simulink model "part_n"  (R2022b)
settings: Solver=ode4  StartTime=0.0  StopTime=inf  FixedStep=0.002  RelTol=1e-3
InitFcn:
  | init; % init script
undefined symbols (not defined in the file or in its folder): attitude_m0, attitude_t0, d_state_m, d_state_t, k_epsilon_lead_angle, k_sigma_lead_angle, state_m0, state_t0
libraries: simulink x1
settings Model: SimulationMode=external  Creator=Ali  LastModifiedBy=Ali
settings HardwareCC: ProdBitPerLong=64  ProdHWDeviceType=Intel->x86-64 (Linux 64)
settings RTWCC: Description=Simulink Desktop Real-Time  SystemTargetFile=sldrt.tlc  TemplateMakefile=sldrt.tmf  RTWCompilerOptimization=on
settings CodeAppCC: MaxIdLength=95
settings SimulinkDesktopRealTimeCC: TargetLibSuffix=_sldrt.a  TargetPreCompLibLocation=/Applications/MATLAB_R2022b.app/toolbox/sldrt/lib/maci64

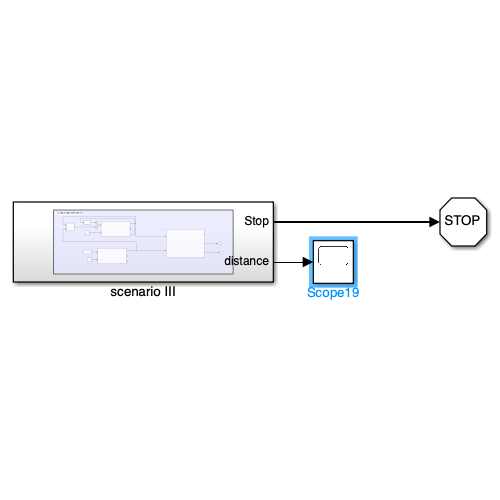
[thumbnail: Simulink's stored preview of the top-level diagram]
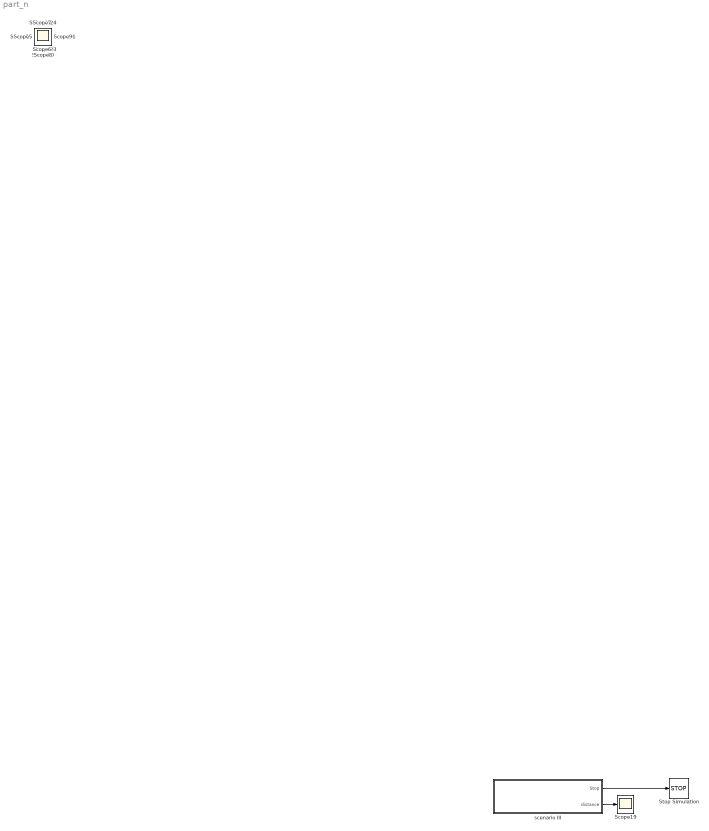
== system part_n ==
  Scope{,1..24} (25 alike) : Scope
  Stop Simulation : Stop
  scenario III : Subsystem
  wires:
  scenario III/1(Stop) -> Stop Simulation/1
  scenario III/2(distance) -> Scope19/1

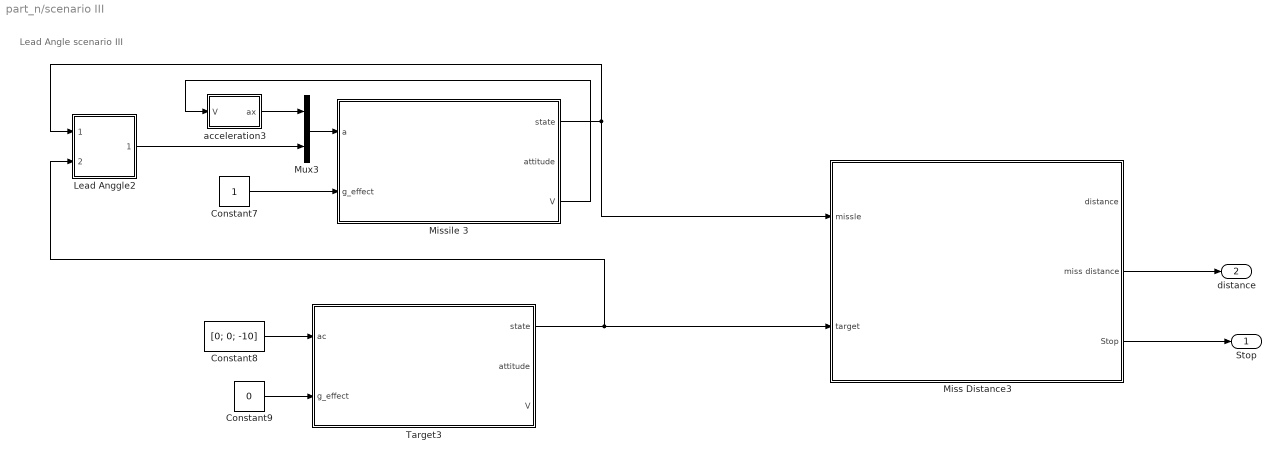
== system part_n/scenario III ==
  note: Lead Angle scenario III
  Constant7 : Constant
  Constant8 : Constant  Value=[0; 0; -10]
  Constant9 : Constant  Value=0
  Lead Anggle2 : Subsystem
  Miss Distance3 : Subsystem
  Missile 3 : Subsystem
  Mux3 : Mux  Inputs=2
  Target3 : Subsystem
  acceleration3 : Subsystem
  Stop : Outport
  distance : Outport  Port=2
  wires:
  Miss Distance3/3(Stop) -> Stop/1
  Target3/1(state) -> Lead Anggle2/2(target_state), Miss Distance3/2(target)
  acceleration3/1(ax) -> Mux3/1
  Lead Anggle2/1("ay, az") -> Mux3/2
  Missile 3/1(state) -> Lead Anggle2/1(missle_state), Miss Distance3/1(missle)
  Constant7/1 -> Missile 3/2(g_effect)
  Constant9/1 -> Target3/2(g_effect)
  Missile 3/3(V) -> acceleration3/1(V)
  Miss Distance3/2(miss distance) -> distance/1
  Constant8/1 -> Target3/1(ac)
  Mux3/1 -> Missile 3/1(a)

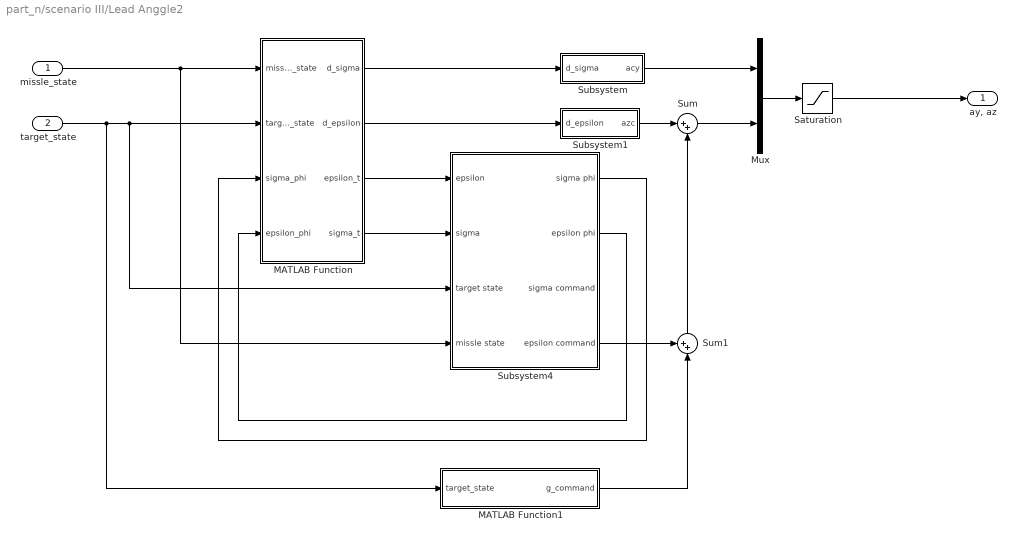
== system part_n/scenario III/Lead Anggle2 ==
  missle_state : Inport
  target_state : Inport  Port=2
  MATLAB Function : MATLAB Function  TreatAsAtomicUnit=on
  MATLAB Function1 : MATLAB Function  TreatAsAtomicUnit=on
  Mux : Mux  Inputs=2
  Saturation : Saturate  UpperLimit=5*9.81  LowerLimit=-5*9.81
  Subsystem : Subsystem
  Subsystem1 : Subsystem
  Subsystem4 : Subsystem
  Sum : Sum  Inputs=|++
  Sum1 : Sum  Inputs=++|
  "ay, az" : Outport
  wires:
  missle_state/1 -> Subsystem4/4(missle state), MATLAB Function/1(missle_state)
  target_state/1 -> MATLAB Function1/1(target_state), Subsystem4/3(target state), MATLAB Function/2(target_state)
  MATLAB Function/1(d_sigma) -> Subsystem/1(d_sigma)
  MATLAB Function/2(d_epsilon) -> Subsystem1/1(d_epsilon)
  Subsystem1/1(azc) -> Sum/1
  Mux/1 -> Saturation/1
  Saturation/1 -> "ay, az"/1
  Subsystem/1(acy) -> Mux/1
  Sum/1 -> Mux/2
  MATLAB Function/3(epsilon_t) -> Subsystem4/1(epsilon)
  MATLAB Function/4(sigma_t) -> Subsystem4/2(sigma)
  Subsystem4/1(sigma phi) -> MATLAB Function/3(sigma_phi)
  Subsystem4/2(epsilon phi) -> MATLAB Function/4(epsilon_phi)
  Sum1/1 -> Sum/2
  MATLAB Function1/1(g_command) -> Sum1/2
  Subsystem4/4(epsilon command) -> Sum1/1

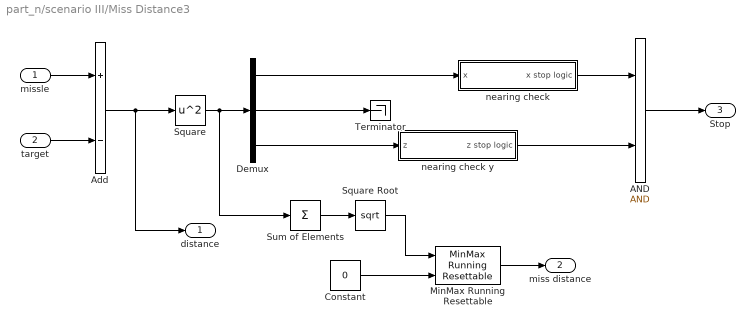
== system part_n/scenario III/Miss Distance3 ==
  missle : Inport
  target : Inport  Port=2
  AND : Logic  IconShape=distinctive  AllPortsSameDT=off  OutDataTypeStr=boolean
  Add : Sum  Inputs=+-
  Constant : Constant  Value=0
  Demux : Demux  Outputs=3
  MinMax Running Resettable : simulink/Math Operations/MinMax Running Resettable  Function=min  vinit=inf
  Square : Math  Operator=square
  Square Root : Sqrt
  Sum of Elements : Sum  Inputs=+
  Terminator : Terminator
  nearing check : Subsystem
  nearing check y : Subsystem
  distance : Outport
  miss distance : Outport  Port=2
  Stop : Outport  Port=3
  wires:
  missle/1 -> Add/1
  Add/1 -> distance/1, Square/1
  target/1 -> Add/2
  Square/1 -> Sum of Elements/1, Demux/1
  nearing check/1(x stop logic) -> AND/1
  AND/1 -> Stop/1
  Demux/2 -> Terminator/1
  nearing check y/1(z stop logic) -> AND/2
  Sum of Elements/1 -> Square Root/1
  Square Root/1 -> MinMax Running Resettable/1
  Demux/3 -> nearing check y/1(z)
  Demux/1 -> nearing check/1(x)
  Constant/1 -> MinMax Running Resettable/2
  MinMax Running Resettable/1 -> miss distance/1

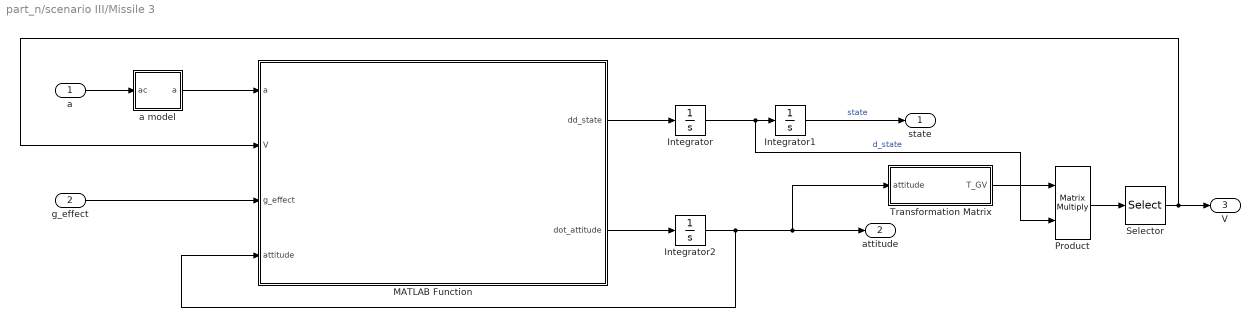
== system part_n/scenario III/Missile 3 ==
  a : Inport
  g_effect : Inport  Port=2
  Integrator : Integrator  InitialCondition=d_state_m
  Integrator1 : Integrator  InitialCondition=state_m0
  Integrator2 : Integrator  InitialCondition=attitude_m0
  MATLAB Function : MATLAB Function  TreatAsAtomicUnit=on
  Product : Product  Multiplication=Matrix(*)
  Selector : Selector  InputPortWidth=3  IndexOptions=Index vector (dialog)  Indices=[1]  OutputSizes=1
  Transformation Matrix : MATLAB Function  TreatAsAtomicUnit=on
  a model : Subsystem
  state : Outport
  attitude : Outport  Port=2
  V : Outport  Port=3
  wires:
  MATLAB Function/2(dot_attitude) -> Integrator2/1
  Integrator1/1 -> state/1  "state"
  MATLAB Function/1(dd_state) -> Integrator/1
  g_effect/1 -> MATLAB Function/3(g_effect)
  Integrator/1 -> Product/2, Integrator1/1  "d_state"
  Product/1 -> Selector/1
  Selector/1 -> MATLAB Function/2(V), V/1
  Transformation Matrix/1(T_GV) -> Product/1
  Integrator2/1 -> Transformation Matrix/1(attitude), attitude/1, MATLAB Function/4(attitude)
  a/1 -> a model/1(ac)
  a model/1(a) -> MATLAB Function/1(a)

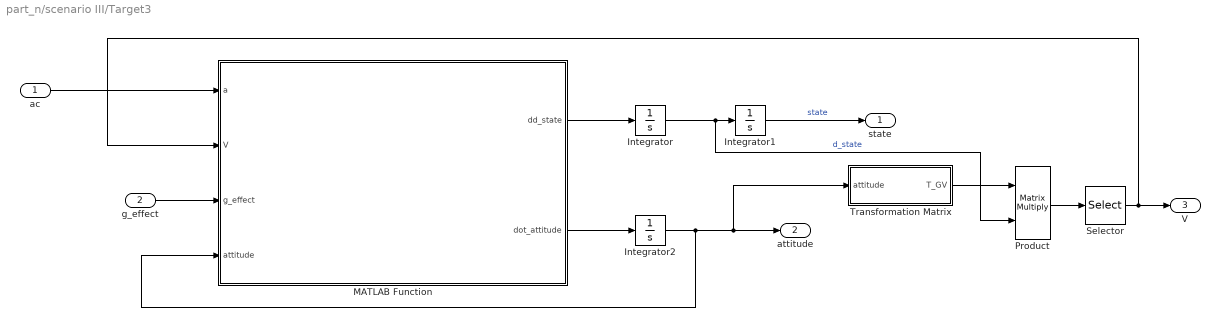
== system part_n/scenario III/Target3 ==
  ac : Inport
  g_effect : Inport  Port=2
  Integrator : Integrator  InitialCondition=d_state_t
  Integrator1 : Integrator  InitialCondition=state_t0
  Integrator2 : Integrator  InitialCondition=attitude_t0
  MATLAB Function : MATLAB Function  TreatAsAtomicUnit=on
  Product : Product  Multiplication=Matrix(*)
  Selector : Selector  InputPortWidth=3  IndexOptions=Index vector (dialog)  Indices=[1]  OutputSizes=1
  Transformation Matrix : MATLAB Function  TreatAsAtomicUnit=on
  state : Outport
  attitude : Outport  Port=2
  V : Outport  Port=3
  wires:
  MATLAB Function/2(dot_attitude) -> Integrator2/1
  Integrator1/1 -> state/1  "state"
  MATLAB Function/1(dd_state) -> Integrator/1
  g_effect/1 -> MATLAB Function/3(g_effect)
  Integrator/1 -> Product/2, Integrator1/1  "d_state"
  Integrator2/1 -> MATLAB Function/4(attitude), Transformation Matrix/1(attitude), attitude/1
  Product/1 -> Selector/1
  Selector/1 -> MATLAB Function/2(V), V/1
  Transformation Matrix/1(T_GV) -> Product/1
  ac/1 -> MATLAB Function/1(a)

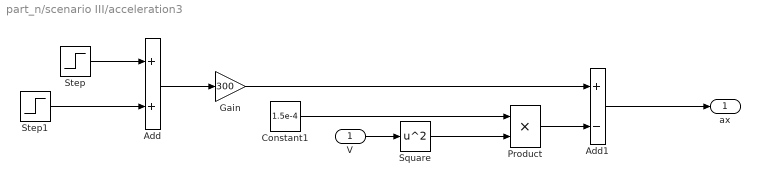
== system part_n/scenario III/acceleration3 ==
  V : Inport
  Add : Sum
  Add1 : Sum  Inputs=+-
  Constant1 : Constant  Value=1.5e-4
  Gain : Gain  Gain=300
  Product : Product
  Square : Math  Operator=square
  Step : Step  Time=3  After=-1  SampleTime=0
  Step1 : Step  Time=0  SampleTime=0
  ax : Outport
  wires:
  V/1 -> Square/1
  Step/1 -> Add/1
  Square/1 -> Product/2
  Constant1/1 -> Product/1
  Add1/1 -> ax/1
  Step1/1 -> Add/2
  Gain/1 -> Add1/1
  Add/1 -> Gain/1
  Product/1 -> Add1/2

== system part_n/scenario III/Lead Anggle2/Subsystem ==
  d_sigma : Inport
  Gain : Gain  Gain=k_sigma_lead_angle
  Sum : Sum  Inputs=+|+
  Transfer Fcn : TransferFcn  Numerator=[1000 0]  Denominator=[1 100]
  acy : Outport
  wires:
  d_sigma/1 -> Gain/1, Transfer Fcn/1
  Transfer Fcn/1 -> Sum/2
  Sum/1 -> acy/1
  Gain/1 -> Sum/1

== system part_n/scenario III/Lead Anggle2/Subsystem1 ==
  d_epsilon : Inport
  Gain1 : Gain  Gain=k_epsilon_lead_angle
  Sum : Sum  Inputs=+|+
  Transfer Fcn : TransferFcn  Numerator=[1000 0]  Denominator=[1 100]
  azc : Outport
  wires:
  d_epsilon/1 -> Transfer Fcn/1, Gain1/1
  Gain1/1 -> Sum/1
  Transfer Fcn/1 -> Sum/2
  Sum/1 -> azc/1

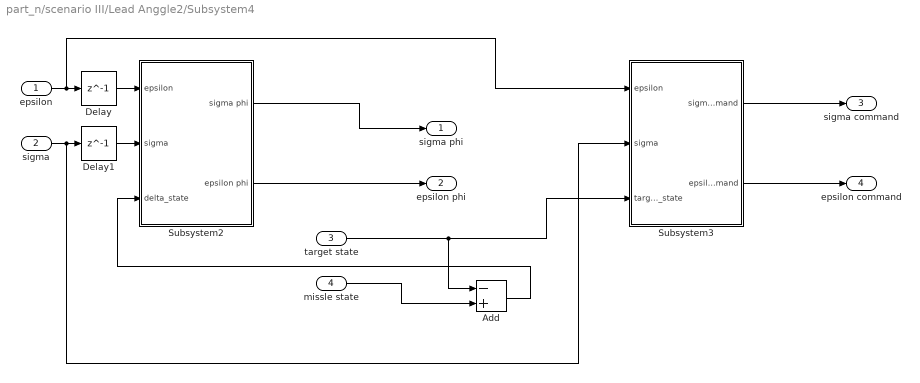
== system part_n/scenario III/Lead Anggle2/Subsystem4 ==
  epsilon : Inport
  sigma : Inport  Port=2
  target state : Inport  Port=3
  missle state : Inport  Port=4
  Add : Sum  Inputs=-+
  Delay : Delay  DelayLength=1
  Delay1 : Delay  DelayLength=1
  Subsystem2 : Subsystem
  Subsystem3 : Subsystem
  sigma phi : Outport
  epsilon phi : Outport  Port=2
  sigma command : Outport  Port=3
  epsilon command : Outport  Port=4
  wires:
  sigma/1 -> Subsystem3/2(sigma), Delay1/1
  epsilon/1 -> Subsystem3/1(epsilon), Delay/1
  Delay1/1 -> Subsystem2/2(sigma)
  Delay/1 -> Subsystem2/1(epsilon)
  Subsystem2/2(epsilon phi) -> epsilon phi/1
  Subsystem2/1(sigma phi) -> sigma phi/1
  target state/1 -> Add/1, Subsystem3/3(target_state)
  missle state/1 -> Add/2
  Add/1 -> Subsystem2/3(delta_state)
  Subsystem3/1(sigma command) -> sigma command/1
  Subsystem3/2(epsilon command) -> epsilon command/1

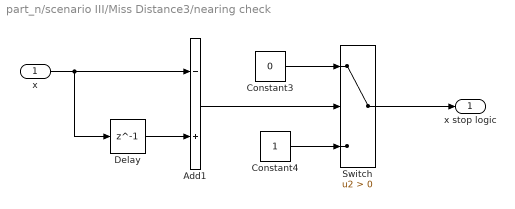
== system part_n/scenario III/Miss Distance3/nearing check ==
  x : Inport
  Add1 : Sum  Inputs=-+
  Constant3 : Constant  Value=0
  Constant4 : Constant
  Delay : Delay  DelayLength=1  InitialCondition=inf
  Switch : Switch  Criteria=u2 > Threshold  SaturateOnIntegerOverflow=off  InputSameDT=off
  x stop logic : Outport
  wires:
  Switch/1 -> x stop logic/1
  Constant3/1 -> Switch/1
  Constant4/1 -> Switch/3
  x/1 -> Delay/1, Add1/1
  Add1/1 -> Switch/2
  Delay/1 -> Add1/2

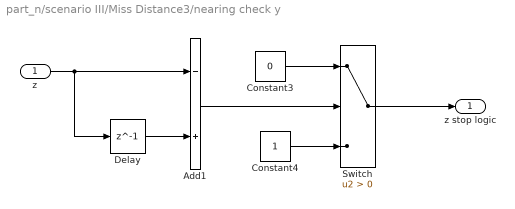
== system part_n/scenario III/Miss Distance3/nearing check y ==
  z : Inport
  Add1 : Sum  Inputs=-+
  Constant3 : Constant  Value=0
  Constant4 : Constant
  Delay : Delay  DelayLength=1  InitialCondition=inf
  Switch : Switch  Criteria=u2 > Threshold  SaturateOnIntegerOverflow=off  InputSameDT=off
  z stop logic : Outport
  wires:
  Delay/1 -> Add1/2
  Add1/1 -> Switch/2
  z/1 -> Add1/1, Delay/1
  Constant4/1 -> Switch/3
  Constant3/1 -> Switch/1
  Switch/1 -> z stop logic/1

== system part_n/scenario III/Missile 3/a model ==
  ac : Inport
  Demux : Demux  Outputs=3
  Mux : Mux  Inputs=3
  Transfer Fcn : TransferFcn  Numerator=[30 200]  Denominator=[1 30 200]
  Transfer Fcn1 : TransferFcn  Numerator=[30 200]  Denominator=[1 30 200]
  a : Outport
  wires:
  Transfer Fcn/1 -> Mux/2
  Mux/1 -> a/1
  Transfer Fcn1/1 -> Mux/3
  Demux/2 -> Transfer Fcn/1
  Demux/3 -> Transfer Fcn1/1
  Demux/1 -> Mux/1
  ac/1 -> Demux/1

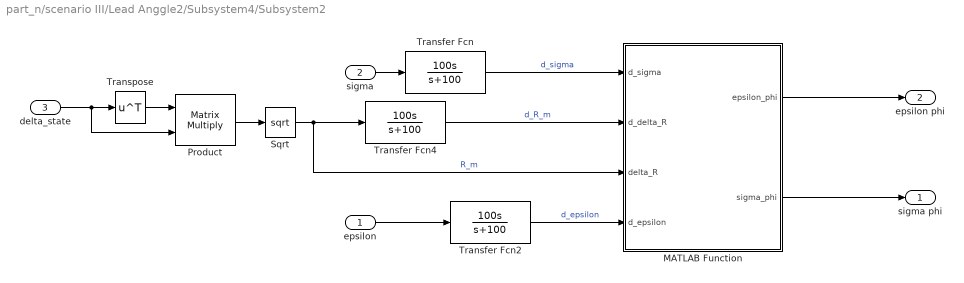
== system part_n/scenario III/Lead Anggle2/Subsystem4/Subsystem2 ==
  epsilon : Inport
  sigma : Inport  Port=2
  delta_state : Inport  Port=3
  MATLAB Function : MATLAB Function  TreatAsAtomicUnit=on
  Product : Product  Multiplication=Matrix(*)
  Sqrt : Sqrt
  Transfer Fcn : TransferFcn  Numerator=[100 0]  Denominator=[1 100]
  Transfer Fcn2 : TransferFcn  Numerator=[100 0]  Denominator=[1 100]
  Transfer Fcn4 : TransferFcn  Numerator=[100 0]  Denominator=[1 100]
  Transpose : Math  Operator=transpose
  sigma phi : Outport
  epsilon phi : Outport  Port=2
  wires:
  sigma/1 -> Transfer Fcn/1
  Transfer Fcn/1 -> MATLAB Function/1(d_sigma)  "d_sigma"
  epsilon/1 -> Transfer Fcn2/1
  Transfer Fcn2/1 -> MATLAB Function/4(d_epsilon)  "d_epsilon"
  delta_state/1 -> Product/2, Transpose/1
  Product/1 -> Sqrt/1
  Transpose/1 -> Product/1
  Sqrt/1 -> MATLAB Function/3(delta_R), Transfer Fcn4/1  "R_m"
  Transfer Fcn4/1 -> MATLAB Function/2(d_delta_R)  "d_R_m"
  MATLAB Function/1(epsilon_phi) -> epsilon phi/1
  MATLAB Function/2(sigma_phi) -> sigma phi/1

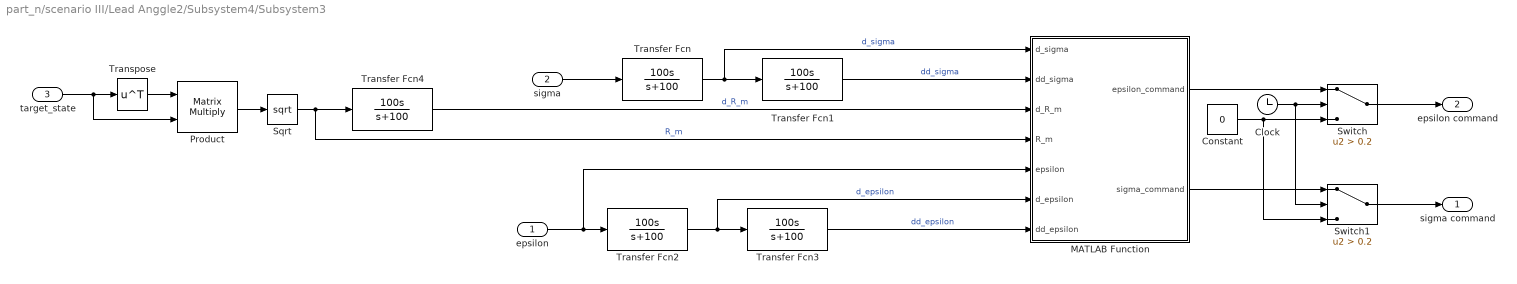
== system part_n/scenario III/Lead Anggle2/Subsystem4/Subsystem3 ==
  epsilon : Inport
  sigma : Inport  Port=2
  target_state : Inport  Port=3
  Clock : Clock
  Constant : Constant  Value=0
  MATLAB Function : MATLAB Function  TreatAsAtomicUnit=on
  Product : Product  Multiplication=Matrix(*)
  Sqrt : Sqrt
  Switch : Switch  Criteria=u2 > Threshold  Threshold=0.2  SaturateOnIntegerOverflow=off  InputSameDT=off
  Switch1 : Switch  Criteria=u2 > Threshold  Threshold=0.2  SaturateOnIntegerOverflow=off  InputSameDT=off
  Transfer Fcn{,1..4} (5 alike) : TransferFcn  Numerator=[100 0]  Denominator=[1 100]
  Transpose : Math  Operator=transpose
  sigma command : Outport
  epsilon command : Outport  Port=2
  wires:
  sigma/1 -> Transfer Fcn/1
  Transfer Fcn1/1 -> MATLAB Function/2(dd_sigma)  "dd_sigma"
  Transfer Fcn/1 -> MATLAB Function/1(d_sigma), Transfer Fcn1/1  "d_sigma"
  epsilon/1 -> MATLAB Function/5(epsilon), Transfer Fcn2/1
  Transfer Fcn2/1 -> MATLAB Function/6(d_epsilon), Transfer Fcn3/1  "d_epsilon"
  target_state/1 -> Product/2, Transpose/1
  Product/1 -> Sqrt/1
  Transpose/1 -> Product/1
  Sqrt/1 -> MATLAB Function/4(R_m), Transfer Fcn4/1  "R_m"
  Transfer Fcn3/1 -> MATLAB Function/7(dd_epsilon)  "dd_epsilon"
  Transfer Fcn4/1 -> MATLAB Function/3(d_R_m)  "d_R_m"
  Clock/1 -> Switch1/2, Switch/2
  Switch/1 -> epsilon command/1
  MATLAB Function/1(epsilon_command) -> Switch/1
  Constant/1 -> Switch1/3, Switch/3
  Switch1/1 -> sigma command/1
  MATLAB Function/2(sigma_command) -> Switch1/1

== matlab function part_n/scenario III/Lead Anggle2/MATLAB Function ==
  data: d_sigma output; missle_state input; d_epsilon output; target_state input; epsilon_t output; sigma_t output; sigma_phi input; epsilon_phi input
function [d_sigma, d_epsilon, epsilon_t, sigma_t] =...
    fcn(missle_state, target_state, sigma_phi, epsilon_phi)

[sigma_m, epsilon_m] = angle_calculator(missle_state);
[sigma_t, epsilon_t] = angle_calculator(target_state);

d_epsilon = norm(missle_state)*(epsilon_t - epsilon_m + epsilon_phi);
d_sigma = norm(missle_state)*(sigma_t - sigma_m + sigma_phi)*cos(epsilon_t+epsilon_phi);

end


function [sigma, epsilon] = angle_calculator(state)
    if norm(state) == 0
        epsilon = 0;
        sigma = 0;
        return
    end
    epsilon = asin(state(3)/norm(state));
    sigma = atan2(state(2),state(1));
end

== matlab function part_n/scenario III/Lead Anggle2/MATLAB Function1 ==
  data: g_command output; target_state input
function g_command  = fcn(target_state)

[~, epsilon_t] = angle_calculator(target_state);
g = 9.81;
g_command = g * cos(epsilon_t);


end


function [sigma, epsilon] = angle_calculator(state)
    if norm(state) == 0
        epsilon = 0;
        sigma = 0;
        return
    end
    epsilon = asin(state(3)/norm(state));
    sigma = atan2(state(2),state(1));
end

== matlab function part_n/scenario III/Lead Anggle2/Subsystem4/Subsystem2/MATLAB Function ==
  data: d_sigma input; d_delta_R input; delta_R input; d_epsilon input; epsilon_phi output; sigma_phi output
function [epsilon_phi, sigma_phi] = fcn(d_sigma, d_delta_R, delta_R, d_epsilon)


t_go = - delta_R / d_delta_R;
epsilon_phi = t_go * d_epsilon;


sigma_phi = t_go * d_sigma;

== matlab function part_n/scenario III/Lead Anggle2/Subsystem4/Subsystem3/MATLAB Function ==
  data: d_sigma input; dd_sigma input; d_R_m input; R_m input; epsilon input; d_epsilon input; dd_epsilon input; epsilon_command output; sigma_command output
function [epsilon_command, sigma_command] = fcn(d_sigma,dd_sigma, d_R_m, R_m, epsilon, d_epsilon, dd_epsilon)


epsilon_command = R_m*dd_epsilon + 2*d_R_m*d_epsilon ...
    + R_m*(d_sigma^2)*sin(epsilon)*cos(epsilon);


sigma_command   = (R_m*dd_sigma + 2*d_R_m*d_sigma)*cos(epsilon) ...
    - 2*R_m*d_epsilon*d_sigma*sin(epsilon);

== matlab function part_n/scenario III/Missile 3/MATLAB Function ==
  data: a input; dd_state output; V input; g_effect input; attitude input; dot_attitude output
function [dd_state, dot_attitude] =...
    fcn(a, V, g_effect, attitude)
a_x = a(1);
a_y = a(2);
a_z = a(3);

theta = attitude(1);
psi = attitude(2);
g = 9.81;
g = g*g_effect;

ddot_x = a_x*cos(theta)*cos(psi) - a_y*sin(psi) - a_z*sin(theta)*cos(psi);
ddot_y = a_x*cos(theta)*sin(psi) + a_y*cos(psi) - a_z*sin(theta)*sin(psi);
ddot_z = a_x*sin(theta) + a_z*cos(theta) - g;

dd_state = [ddot_x; ddot_y; ddot_z];

dot_theta = (a_z - g*cos(theta)) / V;
dot_psi   = a_y / (V*cos(theta));

dot_attitude = [dot_theta; dot_psi];

== matlab function part_n/scenario III/Missile 3/Transformation Matrix ==
  data: attitude input; T_GV output
function T_GV = fcn(attitude)
theta = attitude(1);
psi = attitude(2);

T_GV = [cos(theta)*cos(psi)   cos(theta)*sin(psi)   sin(theta)
            -sin(psi)               cos(psi)            0
        -sin(theta)*cos(psi)  -sin(theta)*sin(psi)   cos(theta) ];

== matlab function part_n/scenario III/Target3/MATLAB Function ==
  data: a input; dd_state output; V input; g_effect input; attitude input; dot_attitude output
function [dd_state, dot_attitude] =...
    fcn(a, V, g_effect, attitude)
a_x = a(1);
a_y = a(2);
a_z = a(3);

theta = attitude(1);
psi = attitude(2);
g = 9.81;
g = g*g_effect;

ddot_x = a_x*cos(theta)*cos(psi) - a_y*sin(psi) - a_z*sin(theta)*cos(psi);
ddot_y = a_x*cos(theta)*sin(psi) + a_y*cos(psi) - a_z*sin(theta)*sin(psi);
ddot_z = a_x*sin(theta) + a_z*cos(theta) - g;


dd_state = [ddot_x; ddot_y; ddot_z];

g = 9.81;
dot_theta = (a_z - g*cos(theta)) / V;
dot_psi   = a_y / (V*cos(theta));

dot_attitude = [dot_theta; dot_psi];

== matlab function part_n/scenario III/Target3/Transformation Matrix ==
  data: attitude input; T_GV output
function T_GV = fcn(attitude)
theta = attitude(1);
psi = attitude(2);

T_GV = [cos(theta)*cos(psi)   cos(theta)*sin(psi)   sin(theta)
            -sin(psi)               cos(psi)            0
        -sin(theta)*cos(psi)  -sin(theta)*sin(psi)   cos(theta) ];
